simulink library "MSP_BDOT_lib"  (R2016b)
settings: Solver=VariableStepAuto  StartTime=0.0  StopTime=10.0  RelTol=1e-3
libraries: bdot_controller_lib x1
settings Model: Creator=taylorreynolds  LastModifiedBy=taylorreynolds

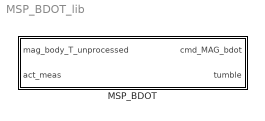
== system MSP_BDOT_lib ==
  MSP_BDOT : Subsystem

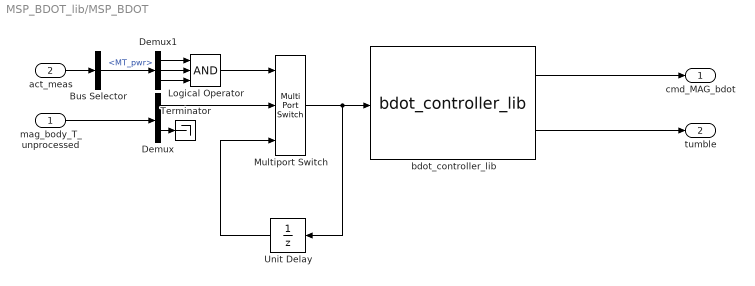
== system MSP_BDOT_lib/MSP_BDOT ==
  mag_body_T_unprocessed : Inport
  act_meas : Inport  Port=2
  Bus Selector : BusSelector  OutputSignals=MT_pwr
  Demux : Demux  Outputs=[3 1]
  Demux1 : Demux  Outputs=3
  Logical Operator : Logic  Inputs=3  AllPortsSameDT=off  OutDataTypeStr=boolean
  Multiport Switch : MultiPortSwitch  DataPortOrder=Zero-based contiguous  Inputs=2
  Terminator : Terminator
  Unit Delay : UnitDelay  SampleTime=-1
  bdot_controller_lib : bdot_controller_lib/bdot_controller_lib
  cmd_MAG_bdot : Outport
  tumble : Outport  Port=2
  wires:
  Unit Delay/1 -> Multiport Switch/3
  Multiport Switch/1 -> bdot_controller_lib/1, Unit Delay/1
  Logical Operator/1 -> Multiport Switch/1
  Demux1/3 -> Logical Operator/3
  Demux1/2 -> Logical Operator/2
  Demux1/1 -> Logical Operator/1
  Bus Selector/1 -> Demux1/1  "<MT_pwr>"
  act_meas/1 -> Bus Selector/1
  bdot_controller_lib/2 -> tumble/1
  bdot_controller_lib/1 -> cmd_MAG_bdot/1
  mag_body_T_unprocessed/1 -> Demux/1
  Demux/2 -> Terminator/1
  Demux/1 -> Multiport Switch/2
